simulink model "swing_up_sim"  (R2021a)
settings: Solver=VariableStepAuto  StartTime=0.0  StopTime=10  FixedStep=0.002  MaxStep=0.0001  RelTol=1e-3
values from neighbouring files (symbols this model uses):
  alpha_0 = 0.0*pi    (= 0)    [swing_up_simulator.m]
  E_r = 2*mp*g*l    [swing_up_simulator.m]
  k_e = 100*Rm/(km*mr*r)    [swing_up_simulator.m]
  K_unstable = lqr(A,B,Q,R)    [unstable_init.m]
undefined symbols (not defined in the file or in its folder): a_max, bp, br, g, Jp, Jr, l, mp, mr, r, tau_max
libraries: simulink x1
settings Model: Creator=willi  LastModifiedBy=magd4814

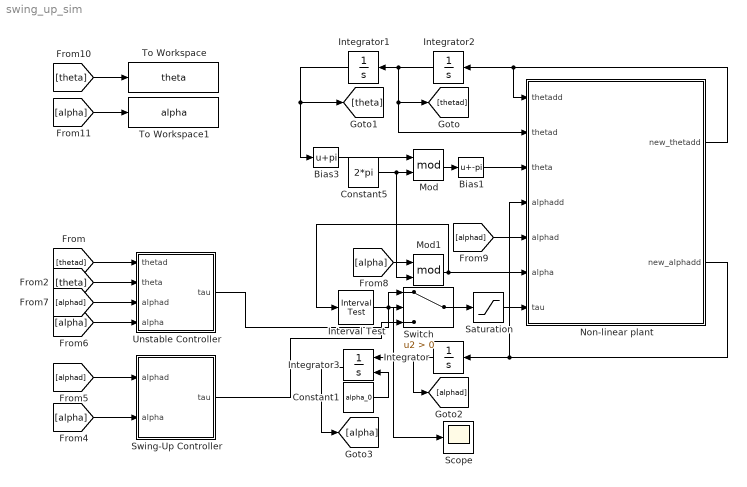
== system swing_up_sim ==
  Bias1 : Bias  Bias=-pi
  Bias3 : Bias  Bias=pi
  Constant1 : Constant  Value=alpha_0
  Constant5 : Constant  Value=2*pi
  Integrator : Integrator
  Integrator1 : Integrator
  Integrator2 : Integrator
  Integrator3 : Integrator  InitialConditionSource=external
  Interval Test : simulink/Logic and Bit Operations/Interval Test  IntervalClosedRight=on  uplimit=1.15*pi  IntervalClosedLeft=on  lowlimit=0.85*pi  OutDataTypeStr=uint8
  Mod : Math  Operator=mod  SaturateOnIntegerOverflow=on
  Mod1 : Math  Operator=mod  SaturateOnIntegerOverflow=on
  Non-linear plant : Subsystem
  Saturation : Saturate  UpperLimit=tau_max  LowerLimit=-tau_max
  Scope : Scope
  Swing-Up Controller : Subsystem
  Switch : Switch  Criteria=u2 > Threshold
  To Workspace : ToWorkspace  VariableName=theta  SaveFormat=Timeseries  SampleTime=-1
  To Workspace1 : ToWorkspace  VariableName=alpha  SaveFormat=Timeseries  SampleTime=-1
  Unstable Controller : Subsystem
  wires:
  Non-linear plant/2(new_alphadd) -> Non-linear plant/4(alphadd), Integrator/1
  Constant1/1 -> Integrator3/2
  Constant5/1 -> Mod1/2, Mod/2
  Mod/1 -> Bias1/1
  Integrator1/1 -> Bias3/1, [theta]
  Bias3/1 -> Mod/1
  Integrator3/1 -> [alpha]
  Bias1/1 -> Non-linear plant/3(theta)
  Integrator/1 -> [alphad], Integrator3/1
  Mod1/1 -> Interval Test/1, Non-linear plant/6(alpha)
  Integrator2/1 -> [thetad], Non-linear plant/2(thetad), Integrator1/1
  Unstable Controller/1(tau) -> Switch/1
  Interval Test/1 -> Scope/1, Switch/2
  [thetad] -> Unstable Controller/1(thetad)
  [theta] -> Unstable Controller/2(theta)
  [alphad] -> Swing-Up Controller/1(alphad)
  [alpha] -> Swing-Up Controller/2(alpha)
  [alphad] -> Unstable Controller/3(alphad)
  [alpha] -> Unstable Controller/4(alpha)
  [alphad] -> Non-linear plant/5(alphad)
  [alpha] -> Mod1/1
  [alpha] -> To Workspace1/1
  [theta] -> To Workspace/1
  Non-linear plant/1(new_thetadd) -> Integrator2/1, Non-linear plant/1(thetadd)
  Switch/1 -> Saturation/1
  Saturation/1 -> Non-linear plant/7(tau)
  Swing-Up Controller/1(tau) -> Switch/3

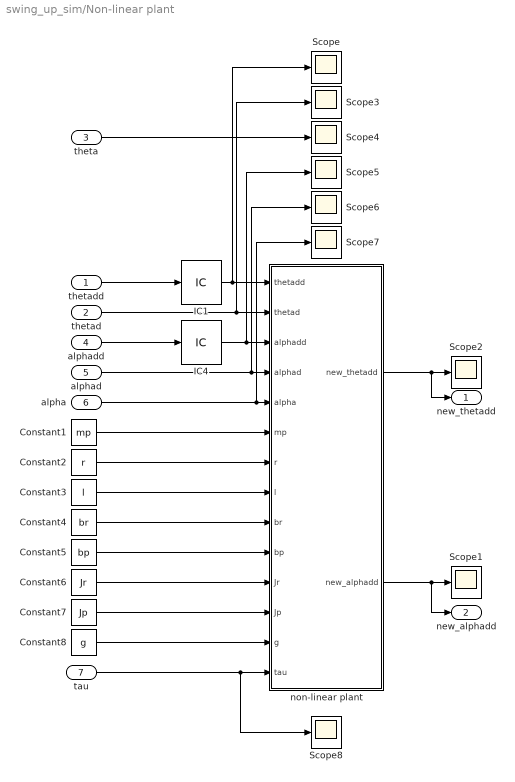
== system swing_up_sim/Non-linear plant ==
  thetadd : Inport
  thetad : Inport  Port=2
  theta : Inport  Port=3
  alphadd : Inport  Port=4
  alphad : Inport  Port=5
  alpha : Inport  Port=6
  tau : Inport  Port=7
  Constant1 : Constant  Value=mp
  Constant2 : Constant  Value=r
  Constant3 : Constant  Value=l
  Constant4 : Constant  Value=br
  Constant5 : Constant  Value=bp
  Constant6 : Constant  Value=Jr
  Constant7 : Constant  Value=Jp
  Constant8 : Constant  Value=g
  IC1 : InitialCondition  Value=0
  IC4 : InitialCondition  Value=0
  Scope{,1..8} (9 alike) : Scope
  non-linear plant : MATLAB Function  TreatAsAtomicUnit=on
  new_thetadd : Outport
  new_alphadd : Outport  Port=2
  wires:
  Constant3/1 -> non-linear plant/8(l)
  Constant2/1 -> non-linear plant/7(r)
  alphad/1 -> Scope6/1, non-linear plant/4(alphad)
  non-linear plant/1(new_thetadd) -> new_thetadd/1, Scope2/1
  alpha/1 -> Scope7/1, non-linear plant/5(alpha)
  Constant1/1 -> non-linear plant/6(mp)
  Constant7/1 -> non-linear plant/12(Jp)
  non-linear plant/2(new_alphadd) -> new_alphadd/1, Scope1/1
  Constant5/1 -> non-linear plant/10(bp)
  theta/1 -> Scope4/1
  Constant4/1 -> non-linear plant/9(br)
  Constant8/1 -> non-linear plant/13(g)
  Constant6/1 -> non-linear plant/11(Jr)
  IC1/1 -> Scope/1, non-linear plant/1(thetadd)
  IC4/1 -> Scope5/1, non-linear plant/3(alphadd)
  thetad/1 -> Scope3/1, non-linear plant/2(thetad)
  thetadd/1 -> IC1/1
  tau/1 -> Scope8/1, non-linear plant/14(tau)
  alphadd/1 -> IC4/1

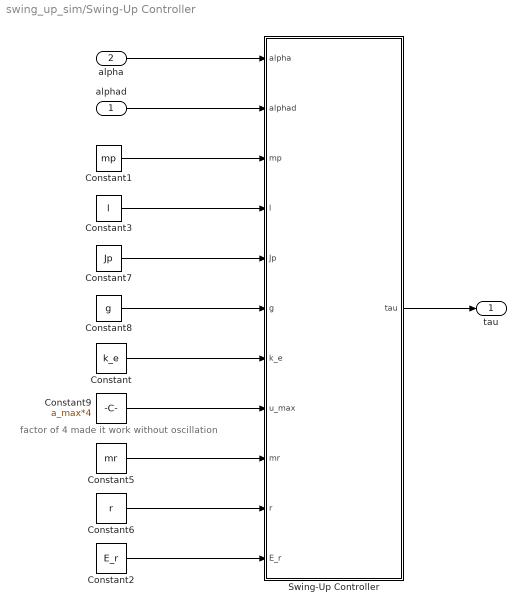
== system swing_up_sim/Swing-Up Controller ==
  note: factor of 4 made it work without oscillation
  alphad : Inport
  alpha : Inport  Port=2
  Constant : Constant  Value=k_e
  Constant1 : Constant  Value=mp
  Constant2 : Constant  Value=E_r
  Constant3 : Constant  Value=l
  Constant5 : Constant  Value=mr
  Constant6 : Constant  Value=r
  Constant7 : Constant  Value=Jp
  Constant8 : Constant  Value=g
  Constant9 : Constant  Value=a_max*4
  Swing-Up Controller : MATLAB Function  TreatAsAtomicUnit=on
  tau : Outport
  wires:
  Constant7/1 -> Swing-Up Controller/5(Jp)
  Constant8/1 -> Swing-Up Controller/6(g)
  Constant1/1 -> Swing-Up Controller/3(mp)
  Constant3/1 -> Swing-Up Controller/4(l)
  Swing-Up Controller/1(tau) -> tau/1
  alphad/1 -> Swing-Up Controller/2(alphad)
  alpha/1 -> Swing-Up Controller/1(alpha)
  Constant/1 -> Swing-Up Controller/7(k_e)
  Constant9/1 -> Swing-Up Controller/8(u_max)
  Constant5/1 -> Swing-Up Controller/9(mr)
  Constant6/1 -> Swing-Up Controller/10(r)
  Constant2/1 -> Swing-Up Controller/11(E_r)

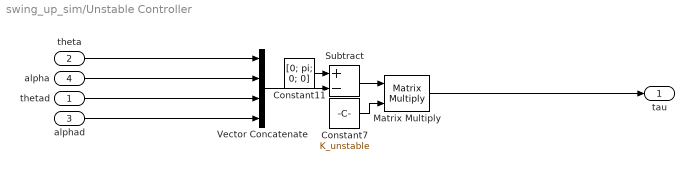
== system swing_up_sim/Unstable Controller ==
  thetad : Inport
  theta : Inport  Port=2
  alphad : Inport  Port=3
  alpha : Inport  Port=4
  Constant11 : Constant  Value=[0; pi; 0; 0]
  Constant7 : Constant  Value=K_unstable
  Matrix Multiply : Product  Multiplication=Matrix(*)
  Subtract : Sum  Inputs=+-
  Vector Concatenate : Concatenate  NumInputs=4
  tau : Outport
  wires:
  thetad/1 -> Vector Concatenate/3
  alpha/1 -> Vector Concatenate/2
  Constant11/1 -> Subtract/1
  Subtract/1 -> Matrix Multiply/1
  Constant7/1 -> Matrix Multiply/2
  theta/1 -> Vector Concatenate/1
  Vector Concatenate/1 -> Subtract/2
  Matrix Multiply/1 -> tau/1
  alphad/1 -> Vector Concatenate/4

== matlab function swing_up_sim/Swing-Up Controller/Swing-Up Controller ==
  data: alpha input; tau output; alphad input; mp input; l input; Jp input; g input; k_e input; u_max input; mr input; r input; E_r input
function tau = fcn(alpha, alphad, mp, l, Jp, g, k_e, u_max, mr, r, E_r)

E = 1/2*Jp*alphad^2 + mp*g*l*(1-cos(alpha));

tau = (mr*r)*u_max*(k_e*(E-E_r)*sign(alphad*cos(alpha)));

== matlab function swing_up_sim/Non-linear plant/non-linear plant ==
  data: thetadd input; thetad input; new_thetadd output; alphadd input; alphad input; alpha input; mp input; r input; l input; br input; bp input; Jr input; Jp input; g input; tau input; new_alphadd output
function [new_thetadd, new_alphadd]= fcn(thetadd, thetad, alphadd, alphad, alpha, mp, r, l, br, bp, Jr, Jp, g, tau)

new_alphadd = (-bp*alphad - mp*g*l*sin(alpha) + Jp*(thetad^2)*sin(alpha)*cos(alpha) - mp*l*r*thetadd*cos(alpha)) / Jp;
new_thetadd = (tau - br*thetad + mp*l*r*(alphad^2)*sin(alpha) - 2*Jp*alphad*thetad*sin(alpha)*cos(alpha) - mp*l*r*alphadd*cos(alpha)) / (Jr+Jp*(sin(alpha)^2));
